simulink model "quad_equation_3d_2024a"  (R2024a)
settings: Solver=VariableStepAuto  StartTime=0.0  StopTime=10  RelTol=1e-3
values from neighbouring files (symbols this model uses):
  b_moment = 0.1    [quad_param_3d.m]
  g = 9.81    [quad_param_3d.m]
  I = [Ixx, 0, 0 ... (first row only)    [quad_param_3d.m]
  k = 0.01    [quad_param_3d.m]
  k_thrust = 0.1    [quad_param_3d.m]
  L = 0.086    [quad_param_3d.m]
  M = 3.3    [quad_param_3d.m]
  Xinit = [0;0;0;0;0;0;0;0;0;0;0;0]    [quad_param_3d.m]
libraries: simulink_extras x1
settings Model: Creator=Admin  LastModifiedBy=Admin

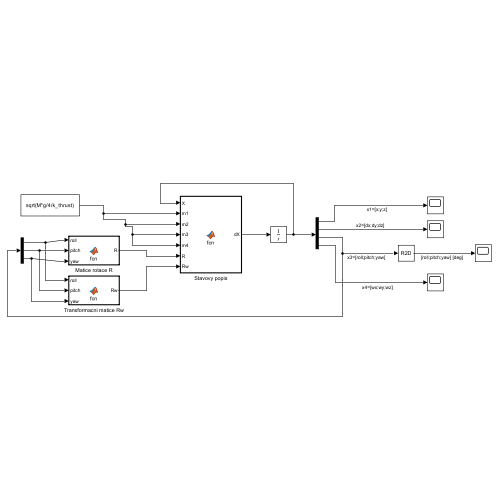
[thumbnail: Simulink's stored preview of the top-level diagram]
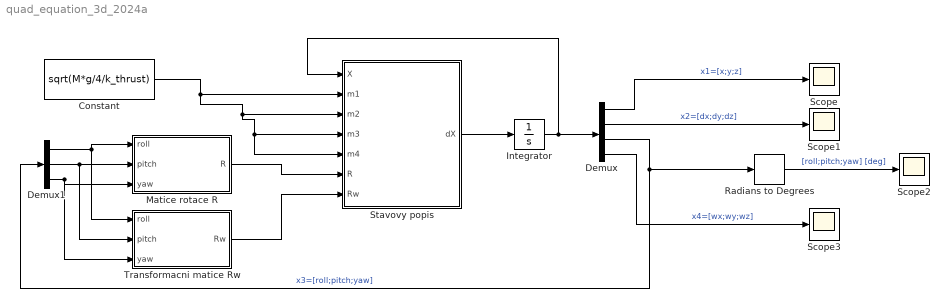
== system quad_equation_3d_2024a ==
  Constant : Constant  Value=sqrt(M*g/4/k_thrust)
  Demux : Demux
  Demux1 : Demux  Outputs=3
  Integrator : Integrator  InitialCondition=Xinit
  Matice rotace R : MATLAB Function  TreatAsAtomicUnit=on
  Radians to Degrees : simulink_extras/Transformations/Radians to Degrees
  Scope{,1..3} (4 alike) : Scope
  Stavovy popis : MATLAB Function  TreatAsAtomicUnit=on
  Transformacni matice Rw : MATLAB Function  TreatAsAtomicUnit=on
  wires:
  Matice rotace R/1(R) -> Stavovy popis/6(R)
  Transformacni matice Rw/1(Rw) -> Stavovy popis/7(Rw)
  Stavovy popis/1(dX) -> Integrator/1
  Integrator/1 -> Stavovy popis/1(X), Demux/1
  Demux/1 -> Scope/1  "x1=[x;y;z]"
  Demux/2 -> Scope1/1  "x2=[dx;dy;dz]"
  Demux/3 -> Radians to Degrees/1, Demux1/1  "x3=[roll;pitch;yaw]"
  Demux/4 -> Scope3/1  "x4=[wx;wy;wz]"
  Constant/1 -> Stavovy popis/5(m4), Stavovy popis/4(m3), Stavovy popis/3(m2), Stavovy popis/2(m1)
  Demux1/1 -> Transformacni matice Rw/1(roll), Matice rotace R/1(roll)
  Demux1/2 -> Matice rotace R/2(pitch), Transformacni matice Rw/2(pitch)
  Demux1/3 -> Transformacni matice Rw/3(yaw), Matice rotace R/3(yaw)
  Radians to Degrees/1 -> Scope2/1  "[roll;pitch;yaw] [deg]"

== matlab function quad_equation_3d_2024a/Matice rotace R ==
  data: roll input; R output; pitch input; yaw input
function R = fcn(roll, pitch, yaw)
% Prepocet matice rotace R=Rx*Ry*Rz

R_x = [1, 0, 0; 
       0, cos(roll), -sin(roll);
       0, sin(roll), cos(roll)];

R_y = [cos(pitch), 0, sin(pitch); 
       0, 1, 0; 
      -sin(pitch), 0, cos(pitch)];

R_z = [cos(yaw), -sin(yaw), 0; 
       sin(yaw), cos(yaw), 0; 
       0, 0, 1];

R = R_x * R_y * R_z;

== matlab function quad_equation_3d_2024a/Stavovy popis ==
  data: X input; m1 input; dX output; m2 input; m3 input; m4 input; R input; Rw input; k_thrust parameter; k parameter; I parameter; g parameter; M parameter; L parameter; b_moment parameter
function dX  = fcn(X, m1, m2, m3, m4, R, Rw, k_thrust, k, I, g, M, L, b_moment)
% m1, m2, m3, m4 jsou odpovidajici uhlove rychlosti rotoru
% Stavovy popis
% x1 - pozice dronu v prostoru, [x;y;z]
% x2 - linearni rychlost, [dx;dy;dz]
% x3 - Eulerove uhly, [roll;pitch;yaw]
% x4 - vektor uhlovych rychlosti, [wx;wy;wz]
x1 = X(1:3);
x2 = X(4:6);
x3 = X(7:9);
x4 = X(10:12);

Thrust = k_thrust*(m1^2 + m2^2 + m3^2 + m4^2); % tahova sila v soustave tela
Friction = -k * x2; % odporova sila v soustave sveta
Tau_roll = L*k_thrust*(m1^2 + m4^2 - m2^2 - m3^2);
Tau_pitch = L*k_thrust*(m4^2 + m3^2 - m1^2 - m2^2);
Tau_yaw = b_moment*(m1^2 + m3^2 - m2^2 - m4^2);

dx1 = x2;
dx2 = [0; 0; -g] + 1/M*R*[0; 0; Thrust] + 1/M*Friction;
dx3 = Rw * x4;
dx4 = I\( [Tau_roll; Tau_pitch; Tau_yaw] -  cross( x4, (I*x4) ) );

dX = [dx1; dx2; dx3; dx4];

== matlab function quad_equation_3d_2024a/Transformacni matice Rw ==
  data: roll input; Rw output; pitch input; yaw input
function Rw = fcn(roll, pitch, yaw)
% Prepocet matice pro transformace derivaci Eulerovych uhlu 
% do uhlove rychlosti v soustave tela
Rw = [1, 0, -sin(pitch);
      0, cos(roll), cos(pitch)*sin(roll);
      0 -sin(roll), cos(pitch)*cos(roll)];
